simulink model "Ford_T3T6_ArchCnctnDigrm"  (R2016b)
settings: Solver=FixedStepDiscrete  StartTime=0.0  StopTime=10.0  RelTol=1e-3  EnableMultiTasking=on
libraries: canmsglib x15
(part 10 of 15)

== system Ford_T3T6_ArchCnctnDigrm/Monitor System/Measured Signals/ADC ==
  note: ASIL D
  CM012A_FordT3McuCfg : Subsystem  Tag=2.1.0  Description=Program specific I/O and Constant settings for the Ford T3 Program
      settings: AttributesFormatString=Version: %<Tag>
  ES251A_BattRtnCurr : Subsystem  Tag=1.1.0  Description=Receives ADC samples and converts them to battery return current levelexpressed in amperes. Current is saturated before outputed.
      settings: AttributesFormatString=Version: %<Tag>
  EcuT : Outport
  BattVltg : Outport  Port=2
  BattVltgSwd1 : Outport  Port=3
  tag scope: Adc1ScanGroup2Ref0=global, Adc1ScanGroup2Ref1=global, Adc1ScanGroup3Ref0=global, Adc1ScanGroup3Ref1=global, Adc1SelfDiag0=global, Adc1SelfDiag2=global, Adc1SelfDiag4=global, BattRtnCurrAdc=global, BattRtnCurrAdcFaild=global, BattRtnCurrAmpr=global, BattRtnCurrStsQlfr=global, BattVltg=global, BattVltgAdcFaild=global, BattVltgSwd1=global, BattVltgSwd1AdcFaild=global, ChrgPmpDiag=global, ChrgPmpDiagAdcFaild=global, EcuT=global, EcuTAdcFaild=global, HwAg1SnsrNr=global, HwAg1SnsrTyp=global, MotAg2Cos=global, MotAg2CosAdcFaild=global, MotAg2Sin=global, MotAg2SinAdcFaild=global, MotAg5CosAdcFaild=global, MotAg5SinAdcFaild=global, MotAg6CosAdcFaild=global, MotAg6SinAdcFaild=global, MotCtrlAdc0ScanGroup2Ref0=global, MotCtrlAdc0ScanGroup2Ref1=global, MotCtrlAdc0ScanGroup3Ref0=global, MotCtrlAdc0ScanGroup3Ref1=global, MotCtrlAdc0SelfDiag0=global, MotCtrlAdc0SelfDiag2=global, MotCtrlAdc0SelfDiag4=global, MotCtrlBattRtnCurrAmprFastLoop=global, MotCtrlMotAg5Cos=global, MotCtrlMotAg5Sin=global, MotCtrlMotAg6Cos=global, MotCtrlMotAg6Sin=global, MotCtrlMotCurrAdcPeakA=global, MotCtrlMotCurrAdcPeakB=global, MotCtrlMotCurrAdcPeakC=global, MotCtrlMotCurrAdcVlyA=global, MotCtrlMotCurrAdcVlyB=global, MotCtrlMotCurrAdcVlyC=global, MotCtrlMotCurrSnsrOffs1=global, MotCurrAdcPeakAAdcFaild=global, MotCurrAdcPeakBAdcFaild=global, MotCurrAdcPeakCAdcFaild=global, MotCurrAdcVlyAAdcFaild=global, MotCurrAdcVlyBAdcFaild=global, MotCurrAdcVlyCAdcFaild=global, MotCurrSnsrOffs1AdcFaild=global, MotDrvr1IninTestCmpl=global, PwrDiscnctSwtDiag=global, PwrDiscnctSwtDiagAdcFaild=global
  wires:
  [Adc0Faild] -> CM012A_FordT3McuCfg/1(Adc0Faild)
  [Adc1Faild] -> CM012A_FordT3McuCfg/2(Adc1Faild)
  [Adc1RawRes] -> CM012A_FordT3McuCfg/3(Adc1RawRes)
  [EcuId] -> CM012A_FordT3McuCfg/4(EcuId)
  [MotCtrlAdc0RawRes] -> CM012A_FordT3McuCfg/5(MotCtrlAdc0RawRes)
  [GetRefTmr1MicroSec32bit] -> CM012A_FordT3McuCfg/6(GetRefTmr1MicroSec32bit)
  [GetTiSpan1MicroSec32bit] -> CM012A_FordT3McuCfg/7(GetTiSpan1MicroSec32bit)
  CM012A_FordT3McuCfg/1(Adc1ScanGroup2Ref0) -> [Adc1ScanGroup2Ref0]
  CM012A_FordT3McuCfg/2(Adc1ScanGroup2Ref1) -> [Adc1ScanGroup2Ref1]
  CM012A_FordT3McuCfg/3(Adc1ScanGroup3Ref0) -> [Adc1ScanGroup3Ref0]
  CM012A_FordT3McuCfg/4(Adc1ScanGroup3Ref1) -> [Adc1ScanGroup3Ref1]
  CM012A_FordT3McuCfg/5(Adc1SelfDiag0) -> [Adc1SelfDiag0]
  CM012A_FordT3McuCfg/6(Adc1SelfDiag2) -> [Adc1SelfDiag2]
  CM012A_FordT3McuCfg/7(Adc1SelfDiag4) -> [Adc1SelfDiag4]
  CM012A_FordT3McuCfg/8(BattRtnCurrAdc) -> [BattRtnCurrAdc]
  CM012A_FordT3McuCfg/9(BattRtnCurrAdcFaild) -> [BattRtnCurrAdcFaild]
  CM012A_FordT3McuCfg/10(BattVltg) -> BattVltg/1, [BattVltg]
  CM012A_FordT3McuCfg/11(BattVltgAdcFaild) -> [BattVltgAdcFaild]
  CM012A_FordT3McuCfg/12(BattVltgSwd1) -> BattVltgSwd1/1, [BattVltgSwd1]
  CM012A_FordT3McuCfg/13(BattVltgSwd1AdcFaild) -> [BattVltgSwd1AdcFaild]
  CM012A_FordT3McuCfg/14(ChrgPmpDiag) -> [ChrgPmpDiag]
  CM012A_FordT3McuCfg/15(ChrgPmpDiagAdcFaild) -> [ChrgPmpDiagAdcFaild]
  CM012A_FordT3McuCfg/16(EcuT) -> EcuT/1, [EcuT]
  CM012A_FordT3McuCfg/17(EcuTAdcFaild) -> [EcuTAdcFaild]
  CM012A_FordT3McuCfg/18(HwAg1SnsrNr) -> [HwAg1SnsrNr]
  CM012A_FordT3McuCfg/19(HwAg1SnsrTyp) -> [HwAg1SnsrTyp]
  CM012A_FordT3McuCfg/20(MotAg2Cos) -> [MotAg2Cos]
  CM012A_FordT3McuCfg/21(MotAg2CosAdcFaild) -> [MotAg2CosAdcFaild]
  CM012A_FordT3McuCfg/22(MotAg2Sin) -> [MotAg2Sin]
  CM012A_FordT3McuCfg/23(MotAg2SinAdcFaild) -> [MotAg2SinAdcFaild]
  CM012A_FordT3McuCfg/24(MotAg5CosAdcFaild) -> [MotAg5CosAdcFaild]
  CM012A_FordT3McuCfg/25(MotAg5SinAdcFaild) -> [MotAg5SinAdcFaild]
  CM012A_FordT3McuCfg/26(MotAg6CosAdcFaild) -> [MotAg6CosAdcFaild]
  CM012A_FordT3McuCfg/27(MotAg6SinAdcFaild) -> [MotAg6SinAdcFaild]
  CM012A_FordT3McuCfg/28(MotCurrAdcPeakAAdcFaild) -> [MotCurrAdcPeakAAdcFaild]
  CM012A_FordT3McuCfg/29(MotCurrAdcPeakBAdcFaild) -> [MotCurrAdcPeakBAdcFaild]
  CM012A_FordT3McuCfg/30(MotCurrAdcPeakCAdcFaild) -> [MotCurrAdcPeakCAdcFaild]
  CM012A_FordT3McuCfg/31(MotCurrAdcVlyAAdcFaild) -> [MotCurrAdcVlyAAdcFaild]
  CM012A_FordT3McuCfg/32(MotCurrAdcVlyBAdcFaild) -> [MotCurrAdcVlyBAdcFaild]
  CM012A_FordT3McuCfg/33(MotCurrAdcVlyCAdcFaild) -> [MotCurrAdcVlyCAdcFaild]
  CM012A_FordT3McuCfg/34(MotCurrSnsrOffs1AdcFaild) -> [MotCurrSnsrOffs1AdcFaild]
  CM012A_FordT3McuCfg/35(PwrDiscnctSwtDiag) -> [PwrDiscnctSwtDiag]
  CM012A_FordT3McuCfg/36(PwrDiscnctSwtDiagAdcFaild) -> [PwrDiscnctSwtDiagAdcFaild]
  CM012A_FordT3McuCfg/37(MotDrvr1IninTestCmpl) -> [MotDrvr1IninTestCmpl]
  CM012A_FordT3McuCfg/38(MotCtrlAdc0ScanGroup2Ref0) -> [MotCtrlAdc0ScanGroup2Ref0]
  CM012A_FordT3McuCfg/39(MotCtrlAdc0ScanGroup2Ref1) -> [MotCtrlAdc0ScanGroup2Ref1]
  CM012A_FordT3McuCfg/40(MotCtrlAdc0ScanGroup3Ref0) -> [MotCtrlAdc0ScanGroup3Ref0]
  CM012A_FordT3McuCfg/41(MotCtrlAdc0ScanGroup3Ref1) -> [MotCtrlAdc0ScanGroup3Ref1]
  CM012A_FordT3McuCfg/42(MotCtrlAdc0SelfDiag0) -> [MotCtrlAdc0SelfDiag0]
  CM012A_FordT3McuCfg/43(MotCtrlAdc0SelfDiag2) -> [MotCtrlAdc0SelfDiag2]
  CM012A_FordT3McuCfg/44(MotCtrlAdc0SelfDiag4) -> [MotCtrlAdc0SelfDiag4]
  CM012A_FordT3McuCfg/45(MotCtrlMotAg5Cos) -> [MotCtrlMotAg5Cos]
  CM012A_FordT3McuCfg/46(MotCtrlMotAg5Sin) -> [MotCtrlMotAg5Sin]
  CM012A_FordT3McuCfg/47(MotCtrlMotAg6Cos) -> [MotCtrlMotAg6Cos]
  CM012A_FordT3McuCfg/48(MotCtrlMotAg6Sin) -> [MotCtrlMotAg6Sin]
  CM012A_FordT3McuCfg/49(MotCtrlMotCurrAdcPeakA) -> [MotCtrlMotCurrAdcPeakA]
  CM012A_FordT3McuCfg/50(MotCtrlMotCurrAdcPeakB) -> [MotCtrlMotCurrAdcPeakB]
  CM012A_FordT3McuCfg/51(MotCtrlMotCurrAdcPeakC) -> [MotCtrlMotCurrAdcPeakC]
  CM012A_FordT3McuCfg/52(MotCtrlMotCurrAdcVlyA) -> [MotCtrlMotCurrAdcVlyA]
  CM012A_FordT3McuCfg/53(MotCtrlMotCurrAdcVlyB) -> [MotCtrlMotCurrAdcVlyB]
  CM012A_FordT3McuCfg/54(MotCtrlMotCurrAdcVlyC) -> [MotCtrlMotCurrAdcVlyC]
  CM012A_FordT3McuCfg/55(MotCtrlMotCurrSnsrOffs1) -> [MotCtrlMotCurrSnsrOffs1]
  [BattRtnCurrAdc] -> ES251A_BattRtnCurr/1(BattRtnCurrAdc)
  [BattRtnCurrAdcFaild] -> ES251A_BattRtnCurr/2(BattRtnCurrAdcFaild)
  [SplyCurrEstim] -> ES251A_BattRtnCurr/3(SplyCurrEstim)
  [SysSt] -> ES251A_BattRtnCurr/4(SysSt)
  [MotCtrlBattRtnCurrAdc] -> ES251A_BattRtnCurr/5(MotCtrlBattRtnCurrAdc)
  [CnvSnpshtData_f32] -> ES251A_BattRtnCurr/6(CnvSnpshtData_f32)
  [CnvSnpshtData_u08] -> ES251A_BattRtnCurr/7(CnvSnpshtData_u08)
  [GetNtcQlfrSts] -> ES251A_BattRtnCurr/8(GetNtcQlfrSts)
  [SetNtcStsAndSnpshtData] -> ES251A_BattRtnCurr/9(SetNtcStsAndSnpshtData)
  ES251A_BattRtnCurr/1(BattRtnCurrAmpr) -> [BattRtnCurrAmpr]
  ES251A_BattRtnCurr/2(BattRtnCurrStsQlfr) -> [BattRtnCurrStsQlfr]
  ES251A_BattRtnCurr/3(MotCtrlBattRtnCurrAmprFastLoop) -> [MotCtrlBattRtnCurrAmprFastLoop]

== system Ford_T3T6_ArchCnctnDigrm/Monitor System/Measured Signals/BatteryVoltage ==
  note: ASIL B
  note: ASIL B
  BattVltg : Inport
  BattVltgSwd1 : Inport  Port=2
  ES250B_BattVltg : Subsystem  Tag=1.1.0  Description=Function produces an output voltage that is used by the software application
      settings: AttributesFormatString=Version: %<Tag>
  ES259B_BattVltgCorrln : Subsystem  Tag=1.4.0  Description=This function does the correlation between the 2 input sensor signals to determine if they are valid.
      settings: AttributesFormatString=Version: %<Tag>
  Terminator : Terminator
  tag scope: BrdgVltg=global, DftBrdgVltgActv=global, SwdVltgLimd=global
  wires:
  ES259B_BattVltgCorrln/2(BattVltgCorrlnIdptSig) -> Terminator/1
  ES259B_BattVltgCorrln/1(BattSwdVltgCorrlnSts) -> ES250B_BattVltg/1(BattSwdVltgCorrlnSts)
  ES250B_BattVltg/1(BrdgVltg) -> [BrdgVltg]
  BattVltg/1 -> ES259B_BattVltgCorrln/1(BattVltg), ES250B_BattVltg/2(BattVltg)
  BattVltgSwd1/1 -> ES250B_BattVltg/3(BattVltgSwd1), ES259B_BattVltgCorrln/3(BattVltgSwd1)
  [DiagcStsIvtr1Inactv] -> ES259B_BattVltgCorrln/5(DiagcStsIvtr1Inactv)
  [FordInhbBattVltgDiagc] -> ES259B_BattVltgCorrln/6(InhbBattVltgDiagc)
  [StrtUpSt] -> ES259B_BattVltgCorrln/7(StrtUpSt)
  [SysSt] -> ES259B_BattVltgCorrln/8(SysSt)
  [GetNtcQlfrSts8] -> ES259B_BattVltgCorrln/9(GetNtcQlfrSts)
  [SetNtcSts8] -> ES259B_BattVltgCorrln/10(SetNtcSts)
  ES259B_BattVltgCorrln/3(DftBrdgVltgActv) -> [DftBrdgVltgActv]
  ES259B_BattVltgCorrln/4(SwdVltgLimd) -> [SwdVltgLimd]
  [BattVltgSwd1AdcFaild] -> ES259B_BattVltgCorrln/4(BattVltgSwd1AdcFaild)
  [BattVltgAdcFaild] -> ES259B_BattVltgCorrln/2(BattVltgAdcFaild)

== system Ford_T3T6_ArchCnctnDigrm/Monitor System/Measured Signals/EcuTemp ==
  note: ASIL B
  EcuT : Inport
  ES210A_EcuTMeas : Subsystem  Tag=4.2.0  Description="Measures and diagnoses an analog based temperature sensor on ECU.  This particular design can tolerate a transfer function that is not necessarily linear but can be interpolated with 8 different XY pairs."
      settings: AttributesFormatString=Version: %<Tag>
  EcuTFild : Outport
  tag scope: DiagcStsLimdTPrfmnc=global, EcuTFild=global
  wires:
  EcuT/1 -> ES210A_EcuTMeas/1(EcuT)
  [EcuTAdcFaild] -> ES210A_EcuTMeas/2(EcuTAdcFaild)
  [CnvSnpshtData_f32] -> ES210A_EcuTMeas/3(CnvSnpshtData_f32)
  [CnvSnpshtData_logl] -> ES210A_EcuTMeas/4(CnvSnpshtData_logl)
  [GetNtcActv8] -> ES210A_EcuTMeas/5(GetNtcActv)
  [SetNtcStsAndSnpshtData8] -> ES210A_EcuTMeas/6(SetNtcStsAndSnpshtData)
  ES210A_EcuTMeas/1(DiagcStsLimdTPrfmnc) -> [DiagcStsLimdTPrfmnc]
  ES210A_EcuTMeas/2(EcuTFild) -> EcuTFild/1, [EcuTFild]

== system Ford_T3T6_ArchCnctnDigrm/Monitor System/Measured Signals/HwAg Signal Measurement and  Arbitration ==
  note: ASIL D
  note: ASIL D
  note: ASIL D
  CM670A_HwAg1Meas : Subsystem  Tag=3.2.1  Description=HandWheel Angle Sensor 1 Measurement Function reads 10th Tooth and 11th Tooth Spur Handwheel angles over SENT and compute absolute Handwheel Angle 1. Function also provides Fault Injection and Trim Manufacturing services
      settings: AttributesFormatString=Version: %<Tag>
  ES238A_HwAgArbn : Subsystem  Tag=2.2.0  Description=Arbitrates handwheel angle channels and provides handwheel angle to the application
      settings: AttributesFormatString=Version: %<Tag>
  ES239A_HwAgCorrln : Subsystem  Tag=2.2.0  Description=Provides signal correlation for handwheel angle per the SSI design.
      settings: AttributesFormatString=Version: %<Tag>
  HwAgMeas : Outport
  HwAgIdptSig : Outport  Port=2
  tag scope: HwAg1AutTrim=global, HwAg1ClrLtch=global, HwAg1ClrTrim=global, HwAg1ReadTrim=global, HwAg1TrimPrfmdSts=global, HwAg1WrTrim=global, HwAgMeas=global
  wires:
  [HwAgAPolarity] -> CM670A_HwAg1Meas/1(HwAg1Polarity)
  [HwAg1SnsrTyp] -> CM670A_HwAg1Meas/2(HwAg1SnsrTyp)
  [CnvSnpshtData_f32] -> CM670A_HwAg1Meas/3(CnvSnpshtData_f32)
  [CnvSnpshtData_u08] -> CM670A_HwAg1Meas/4(CnvSnpshtData_u08)
  [FltInj_u08] -> CM670A_HwAg1Meas/5(FltInj_u08)
  [GetNtcQlfrSts] -> CM670A_HwAg1Meas/6(GetNtcQlfrSts)
  [GetRefTmr1MicroSec32bit] -> CM670A_HwAg1Meas/7(GetRefTmr1MicroSec32bit)
  [GetTiSpan1MicroSec32bit] -> CM670A_HwAg1Meas/8(GetTiSpan1MicroSec32bit)
  [NvMProxy_GetErrorStatus] -> CM670A_HwAg1Meas/9(HwAg1IfFltLtch_GetErrorStatus)
  [NvMProxy_SetRamBlockStatus] -> CM670A_HwAg1Meas/10(HwAg1IfFltLtch_SetRamBlockStatus)
  [NvMProxy_GetErrorStatus] -> CM670A_HwAg1Meas/11(HwAg1Offs_GetErrorStatus)
  [NvMProxy_SetRamBlockStatus] -> CM670A_HwAg1Meas/12(HwAg1Offs_SetRamBlockStatus)
  [IoHwAb_SetFctPrphlHwAg1] -> CM670A_HwAg1Meas/13(IoHwAb_SetFctPrphlHwAg1)
  [SetNtcStsAndSnpshtData10] -> CM670A_HwAg1Meas/14(SetNtcStsAndSnpshtData)
  CM670A_HwAg1Meas/4(HwAg1AutTrim) -> [HwAg1AutTrim]
  CM670A_HwAg1Meas/5(HwAg1ClrLtch) -> [HwAg1ClrLtch]
  CM670A_HwAg1Meas/6(HwAg1ClrTrim) -> [HwAg1ClrTrim]
  CM670A_HwAg1Meas/7(HwAg1ReadTrim) -> [HwAg1ReadTrim]
  CM670A_HwAg1Meas/8(HwAg1TrimPrfmdSts) -> [HwAg1TrimPrfmdSts]
  CM670A_HwAg1Meas/9(HwAg1WrTrim) -> [HwAg1WrTrim]
  CM670A_HwAg1Meas/3(HwAg1RollgCntr) -> ES238A_HwAgArbn/3(HwAgAQlfr), ES239A_HwAgCorrln/4(HwAgARollgCntr)
  [HwAgARollgCntr] -> ES238A_HwAgArbn/4(HwAgARollgCntr)
  [HwAgB] -> ES238A_HwAgArbn/5(HwAgB)
  [HwAgBQlfr] -> ES238A_HwAgArbn/6(HwAgBQlfr)
  [HwAgBRollgCntr] -> ES238A_HwAgArbn/7(HwAgBRollgCntr)
  [FltInj_f32] -> ES238A_HwAgArbn/9(FltInj_f32)
  ES238A_HwAgArbn/1(HwAg) -> HwAgMeas/1, [HwAgMeas]
  [HwAg1SnsrNr] -> ES239A_HwAgCorrln/1(HwAg1SnsrNr)
  CM670A_HwAg1Meas/1(HwAg1) -> ES238A_HwAgArbn/1(HwAg1SnsrNr), ES239A_HwAgCorrln/2(HwAgA)
  CM670A_HwAg1Meas/2(HwAg1Qlfr) -> ES238A_HwAgArbn/2(HwAgA), ES239A_HwAgCorrln/3(HwAgAQlfr)
  [HwAgB] -> ES239A_HwAgCorrln/5(HwAgB)
  [HwAgBQlfr] -> ES239A_HwAgCorrln/6(HwAgBQlfr)
  [HwAgBRollgCntr] -> ES239A_HwAgCorrln/7(HwAgBRollgCntr)
  [FltInj_u08] -> ES239A_HwAgCorrln/8(FltInj_u08)
  [GetNtcQlfrSts] -> ES239A_HwAgCorrln/9(GetNtcQlfrSts)
  [SetNtcSts] -> ES239A_HwAgCorrln/10(SetNtcSts)
  ES239A_HwAgCorrln/1(HwAgCorrlnSt) -> ES238A_HwAgArbn/8(HwAgCorrlnSt)
  ES239A_HwAgCorrln/2(HwAgIdptSig) -> HwAgIdptSig/1

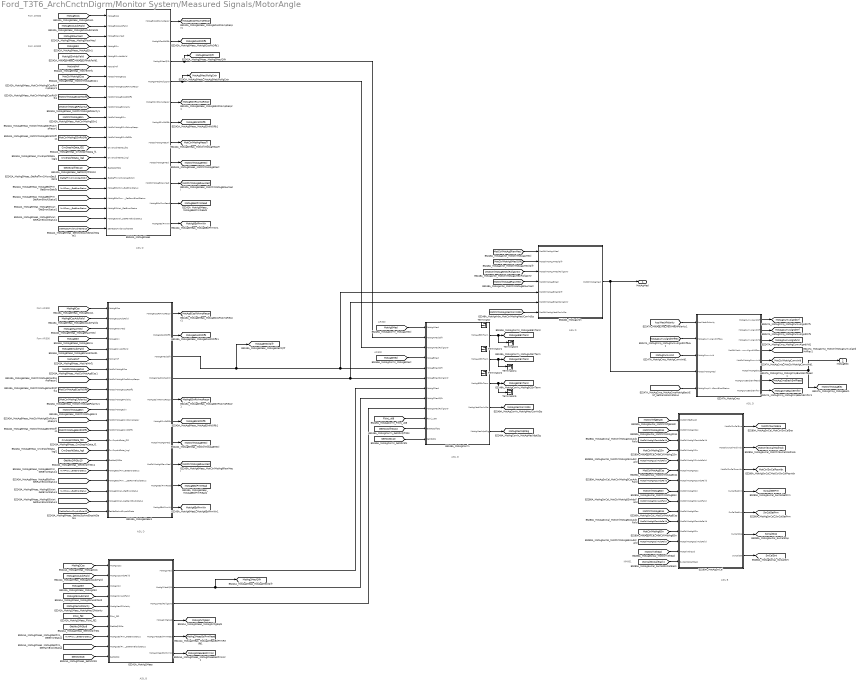
== system Ford_T3T6_ArchCnctnDigrm/Monitor System/Measured Signals/MotorAngle ==
  note: AR300
  note: Fom AR300
  note: ASIL D
  note: ASIL D
  note: ASIL B
  note: ASIL D
  note: ASIL D
  note: ASIL D
  note: ASIL B
  note: Fom AR300
  note: Fom AR300
  note: Fom AR300
  note: AR300
  note: NM001
  ES241A_MotAg2Meas : Subsystem  Tag=1.10.0  Description=This function is responsible for providing a qualified, tertiary motor angle measurement using a sine / cosine based analog sensor
      settings: AttributesFormatString=Version: %<Tag>
  ES242A_MotAg5Meas : Subsystem  Tag=1.3.0  Description=MotAg5Meas funtion shall compute motor angle from Sine and Cosine ADC signals
      settings: AttributesFormatString=Version: %<Tag>
  ES243A_MotAg6Meas1 : Subsystem  Tag=1.4.0  Description=MotAg6Meas funtion shall compute motor angle from Sine and Cosine ADC signals
      settings: AttributesFormatString=Version: %<Tag>
  ES247A_MotAgCmp : Subsystem  Tag=1.8.0  Description=Compensates motor angle for Back EMF and computes cumulative position
      settings: AttributesFormatString=Version: %<Tag>
  ES248A_MotAgArbn : Subsystem  Tag=1.3.0  Description="This function will arbitrate between to motor angle measurements in the motor control loop.  This design assumes that motor angle A is the primary sensor and will use it when possible."
      settings: AttributesFormatString=Version: %<Tag>
  ES249A_MotAgCorrln : Subsystem  Tag=5.0.0  Description=Performs cross check of available motor angle signals. This is necessary for the loss of assist mitigation strategies
      settings: AttributesFormatString=Version: %<Tag>
  ES280A_MotAgSwCal : Subsystem  Tag=2.1.0  Description=Motor Angle Software Calibration
      settings: AttributesFormatString=Version: %<Tag>
  Terminator{,1..5} (6 alike) : Terminator
  MotAgMecl : Outport
  MotAgElec : Outport  Port=2
  tag scope: MotAg2MeasEolPrmRead=global, MotAg2MeasEolPrmWr=global, MotAg2MeclQlfr=global, MotAg2VltgSqd=global, MotAg5CosRtAmpRecpr=global, MotAg5CosRtOffs=global, MotAg5EolPrmRead=global, MotAg5EolPrmWr=global, MotAg5MeclQlfr=global, MotAg5MeclRollgCntr=global, MotAg5SinRtAmpRecpr=global, MotAg5SinRtOffs=global, MotAg6CosRtAmpRecpr=global, MotAg6CosRtOffs=global, MotAg6EolPrmRead=global, MotAg6EolPrmWr=global, MotAg6MeclQlfr=global, MotAg6SinRtAmpRecpr=global, MotAg6SinRtOffs=global, MotAgABErrTerm=global, MotAgACErrTerm=global, MotAgBCErrTerm=global, MotAgCmpBackEmfRead=global, MotAgCmpBackEmfWr=global, MotAgCumvAlgndCrf=global, MotAgCumvAlgndMrf=global, MotAgCumvAlgndVld=global, MotAgMeclCorrlnSts=global, MotAgMeclIdptSig=global, MotCtrlMotAg5Mecl=global, MotCtrlMotAg5RawMecl=global, MotCtrlMotAg6Mecl=global, MotCtrlMotAg6RawMecl=global, MotCtrlMotAgCumvAlgndMrfRev=global, MotCtrlMotAgCumvInid=global, MotCtrlMotAgElec=global, MotCtrlMotAgMeasTi=global, MotCtrlSwCalEna=global, MotCtrlSwCalModlnIdx=global, MotCtrlSwCalPosnIdx=global, SwCalGetPrm=global, SwCalSetPrm=global, SwCalStop=global, SwCalStrt=global
  wires:
  ES247A_MotAgCmp/6(MotCtrlMotAgElec) -> MotAgElec/1, [MotCtrlMotAgElec]
  ES243A_MotAg6Meas1/3(MotAg6MeclQlfr) -> [MotAg6MeclQlfr], ES249A_MotAgCorrln/5(MotAgBMeclQlfr), ES248A_MotAgArbn/5(MotCtrlMotAgBMeclQlfr)
  ES243A_MotAg6Meas1/4(MotAg6MeclRollgCntr) -> ES249A_MotAgCorrln/6(MotAgBMeclRollgCntr), ES248A_MotAgArbn/6(MotCtrlMotAgBMeclRollgCntr)
  ES242A_MotAg5Meas/4(MotAg5MeclRollgCntr) -> [MotAg5MeclRollgCntr], ES249A_MotAgCorrln/3(MotAgAMeclRollgCntr)
  ES242A_MotAg5Meas/3(MotAg5MeclQlfr) -> [MotAg5MeclQlfr], ES249A_MotAgCorrln/2(MotAgAMeclQlfr)
  ES241A_MotAg2Meas/1(MotAg2Mecl) -> ES249A_MotAgCorrln/7(MotAgCMecl)
  ES241A_MotAg2Meas/2(MotAg2MeclQlfr) -> [MotAg2MeclQlfr], ES249A_MotAgCorrln/8(MotAgCMeclQlfr)
  ES241A_MotAg2Meas/3(MotAg2MeclRollgCntr) -> ES249A_MotAgCorrln/9(MotAgCMeclRollgCntr)
  [MotCtrlMfgEnaSt] -> ES280A_MotAgSwCal/1(MotCtrlMfgEnaSt)
  [MotCtrlMotAg2Cos] -> ES280A_MotAgSwCal/2(MotCtrlMotAg2Cos)
  [MotCtrlMotAg2CosAdcFaild] -> ES280A_MotAgSwCal/3(MotCtrlMotAg2CosAdcFaild)
  [MotCtrlMotAg2Sin] -> ES280A_MotAgSwCal/4(MotCtrlMotAg2Sin)
  [MotCtrlMotAg2SinAdcFaild] -> ES280A_MotAgSwCal/5(MotCtrlMotAg2SinAdcFaild)
  [MotCtrlMotAg5Cos] -> ES280A_MotAgSwCal/6(MotCtrlMotAg5Cos)
  [MotCtrlMotAg5CosAdcFaild] -> ES280A_MotAgSwCal/7(MotCtrlMotAg5CosAdcFaild)
  [MotCtrlMotAg5Sin] -> ES280A_MotAgSwCal/8(MotCtrlMotAg5Sin)
  [MotCtrlMotAg5SinAdcFaild] -> ES280A_MotAgSwCal/9(MotCtrlMotAg5SinAdcFaild)
  [MotCtrlMotAg6Cos] -> ES280A_MotAgSwCal/10(MotCtrlMotAg6Cos)
  [MotCtrlMotAg6CosAdcFaild] -> ES280A_MotAgSwCal/11(MotCtrlMotAg6CosAdcFaild)
  [MotCtrlMotAg6Sin] -> ES280A_MotAgSwCal/12(MotCtrlMotAg6Sin)
  [MotCtrlMotAg6SinAdcFaild] -> ES280A_MotAgSwCal/13(MotCtrlMotAg6SinAdcFaild)
  [MotCtrlVehSpd] -> ES280A_MotAgSwCal/14(MotCtrlVehSpd)
  [SwCalStsCallBack] -> ES280A_MotAgSwCal/15(SwCalStsCallBack)
  ES280A_MotAgSwCal/1(MotCtrlSwCalEna) -> [MotCtrlSwCalEna]
  ES280A_MotAgSwCal/2(MotCtrlSwCalModlnIdx) -> [MotCtrlSwCalModlnIdx]
  ES280A_MotAgSwCal/3(MotCtrlSwCalPosnIdx) -> [MotCtrlSwCalPosnIdx]
  ES280A_MotAgSwCal/4(SwCalGetPrm) -> [SwCalGetPrm]
  ES280A_MotAgSwCal/5(SwCalSetPrm) -> [SwCalSetPrm]
  ES280A_MotAgSwCal/6(SwCalStop) -> [SwCalStop]
  ES280A_MotAgSwCal/7(SwCalStrt) -> [SwCalStrt]
  [FltInj_u08] -> ES249A_MotAgCorrln/10(FltInj_u08)
  [GetNtcQlfrSts10] -> ES249A_MotAgCorrln/11(GetNtcQlfrSts)
  [SetNtcSts10] -> ES249A_MotAgCorrln/12(SetNtcSts)
  ES249A_MotAgCorrln/1(MotAgABErrTerm) -> Terminator3/1, [MotAgABErrTerm]
  ES249A_MotAgCorrln/2(MotAgACErrTerm) -> Terminator4/1, [MotAgACErrTerm]
  ES249A_MotAgCorrln/3(MotAgBCErrTerm) -> Terminator5/1, [MotAgBCErrTerm]
  ES249A_MotAgCorrln/5(MotAgMeclIdptSig) -> [MotAgMeclIdptSig]
  [MotAg2Cos] -> ES241A_MotAg2Meas/1(MotAg2Cos)
  [MotAg2CosAdcFaild] -> ES241A_MotAg2Meas/2(MotAg2CosAdcFaild)
  [MotAg2Sin] -> ES241A_MotAg2Meas/3(MotAg2Sin)
  [MotAg2SinAdcFaild] -> ES241A_MotAg2Meas/4(MotAg2SinAdcFaild)
  [MotAgMeclAPolarity] -> ES241A_MotAg2Meas/5(MotAgMecl2Polarity)
  [FltInj_f32] -> ES241A_MotAg2Meas/6(FltInj_f32)
  [GetNtcQlfrSts8] -> ES241A_MotAg2Meas/7(GetNtcQlfrSts)
  [NvMProxy_GetErrorStatus] -> ES241A_MotAg2Meas/8(MotAg2EolPrm_GetErrorStatus)
  [NvMProxy_SetRamBlockStatus] -> ES241A_MotAg2Meas/9(MotAg2EolPrm_SetRamBlockStatus)
  [SetNtcSts8] -> ES241A_MotAg2Meas/10(SetNtcSts)
  ES241A_MotAg2Meas/4(MotAg2VltgSqd) -> [MotAg2VltgSqd]
  ES241A_MotAg2Meas/5(MotAg2MeasEolPrmRead) -> [MotAg2MeasEolPrmRead]
  ES241A_MotAg2Meas/6(MotAg2MeasEolPrmWr) -> [MotAg2MeasEolPrmWr]
  [MotAg5Cos] -> ES242A_MotAg5Meas/1(MotAg5Cos)
  [MotAg5CosAdcFaild] -> ES242A_MotAg5Meas/2(MotAg5CosAdcFaild)
  [MotAg0RawMecl] -> ES242A_MotAg5Meas/3(MotAg5RawMecl)
  [MotAg5Sin] -> ES242A_MotAg5Meas/4(MotAg5Sin)
  [MotAg5SinAdcFaild] -> ES242A_MotAg5Meas/5(MotAg5SinAdcFaild)
  [MotVelMrf] -> ES242A_MotAg5Meas/6(MotVelMrf)
  [MotCtrlMotAg5Cos] -> ES242A_MotAg5Meas/7(MotCtrlMotAg5Cos)
  [MotCtrlMotAg5CosRtAmpRecpr] -> ES242A_MotAg5Meas/8(MotCtrlMotAg5CosRtAmpRecpr)
  [MotCtrlMotAg5CosRtOffs] -> ES242A_MotAg5Meas/9(MotCtrlMotAg5CosRtOffs)
  [MotCtrlMotAgBPolarity] -> ES242A_MotAg5Meas/10(MotCtrlMotAg5Polarity)
  [MotCtrlMotAg5Sin] -> ES242A_MotAg5Meas/11(MotCtrlMotAg5Sin)
  [MotCtrlMotAg5SinRtAmpRecpr] -> ES242A_MotAg5Meas/12(MotCtrlMotAg5SinRtAmpRecpr)
  [MotCtrlMotAg5SinRtOffs] -> ES242A_MotAg5Meas/13(MotCtrlMotAg5SinRtOffs)
  [CnvSnpshtData_f32] -> ES242A_MotAg5Meas/14(CnvSnpshtData_f32)
  [CnvSnpshtData_logl] -> ES242A_MotAg5Meas/15(CnvSnpshtData_logl)
  [GetNtcQlfrSts10] -> ES242A_MotAg5Meas/16(GetNtcQlfrSts)
  [GetRefTmr1MicroSec32bit] -> ES242A_MotAg5Meas/17(GetRefTmr1MicroSec32bit)
  [NvMProxy_GetErrorStatus] -> ES242A_MotAg5Meas/18(MotAg5EolPrm_GetErrorStatus)
  [NvMProxy_SetRamBlockStatus] -> ES242A_MotAg5Meas/19(MotAg5EolPrm_SetRamBlockStatus)
  [NvMProxy_GetErrorStatus] -> ES242A_MotAg5Meas/20(MotAg5StVari_GetErrorStatus)
  [NvMProxy_SetRamBlockStatus] -> ES242A_MotAg5Meas/21(MotAg5StVari_SetRamBlockStatus)
  [SetNtcStsAndSnpshtData10] -> ES242A_MotAg5Meas/22(SetNtcStsAndSnpshtData)
  ES242A_MotAg5Meas/1(MotAg5CosRtAmpRecpr) -> [MotAg5CosRtAmpRecpr]
  ES242A_MotAg5Meas/2(MotAg5CosRtOffs) -> [MotAg5CosRtOffs]
  ES242A_MotAg5Meas/5(MotAg5SinRtAmpRecpr) -> [MotAg5SinRtAmpRecpr]
  ES242A_MotAg5Meas/6(MotAg5SinRtOffs) -> [MotAg5SinRtOffs]
  ES242A_MotAg5Meas/7(MotCtrlMotAgMeasTi) -> [MotCtrlMotAgMeasTi]
  ES242A_MotAg5Meas/8(MotCtrlMotAg5Mecl) -> [MotCtrlMotAg5Mecl]
  ES242A_MotAg5Meas/10(MotAg5EolPrmRead) -> [MotAg5EolPrmRead]
  ES242A_MotAg5Meas/11(MotAg5EolPrmWr) -> [MotAg5EolPrmWr]
  [MotAg6Cos] -> ES243A_MotAg6Meas1/1(MotAg6Cos)
  [MotAg6CosAdcFaild] -> ES243A_MotAg6Meas1/2(MotAg6CosAdcFaild)
  [MotAg1RawMecl] -> ES243A_MotAg6Meas1/3(MotAg6RawMecl)
  [MotAg6Sin] -> ES243A_MotAg6Meas1/4(MotAg6Sin)
  [MotAg6SinAdcFaild] -> ES243A_MotAg6Meas1/5(MotAg6SinAdcFaild)
  [MotVelMrf] -> ES243A_MotAg6Meas1/6(MotVelMrf)
  [MotCtrlMotAg6Cos] -> ES243A_MotAg6Meas1/7(MotCtrlMotAg6Cos)
  [MotCtrlMotAg6CosRtAmpRecpr] -> ES243A_MotAg6Meas1/8(MotCtrlMotAg6CosRtAmpRecpr)
  [MotCtrlMotAg6CosRtOffs] -> ES243A_MotAg6Meas1/9(MotCtrlMotAg6CosRtOffs)
  [MotCtrlMotAgCPolarity] -> ES243A_MotAg6Meas1/10(MotCtrlMotAg6Polarity)
  [MotCtrlMotAg6Sin] -> ES243A_MotAg6Meas1/11(MotCtrlMotAg6Sin)
  [MotCtrlMotAg6SinRtAmpRecpr] -> ES243A_MotAg6Meas1/12(MotCtrlMotAg6SinRtAmpRecpr)
  [MotCtrlMotAg6SinRtOffs] -> ES243A_MotAg6Meas1/13(MotCtrlMotAg6SinRtOffs)
  [CnvSnpshtData_f32] -> ES243A_MotAg6Meas1/14(CnvSnpshtData_f32)
  [CnvSnpshtData_logl] -> ES243A_MotAg6Meas1/15(CnvSnpshtData_logl)
  [GetNtcQlfrSts10] -> ES243A_MotAg6Meas1/16(GetNtcQlfrSts)
  [NvMProxy_GetErrorStatus] -> ES243A_MotAg6Meas1/17(MotAg6EolPrm_GetErrorStatus)
  [NvMProxy_SetRamBlockStatus] -> ES243A_MotAg6Meas1/18(MotAg6EolPrm_SetRamBlockStatus)
  [NvMProxy_GetErrorStatus] -> ES243A_MotAg6Meas1/19(MotAg6StVari_GetErrorStatus)
  [NvMProxy_SetRamBlockStatus] -> ES243A_MotAg6Meas1/20(MotAg6StVari_SetRamBlockStatus)
  [SetNtcStsAndSnpshtData10] -> ES243A_MotAg6Meas1/21(SetNtcStsAndSnpshtData)
  ES243A_MotAg6Meas1/1(MotAg6CosRtAmpRecpr) -> [MotAg6CosRtAmpRecpr]
  ES243A_MotAg6Meas1/2(MotAg6CosRtOffs) -> [MotAg6CosRtOffs]
  ES243A_MotAg6Meas1/5(MotAg6SinRtAmpRecpr) -> [MotAg6SinRtAmpRecpr]
  ES243A_MotAg6Meas1/6(MotAg6SinRtOffs) -> [MotAg6SinRtOffs]
  ES243A_MotAg6Meas1/7(MotCtrlMotAg6Mecl) -> [MotCtrlMotAg6Mecl]
  ES243A_MotAg6Meas1/9(MotAg6EolPrmRead) -> [MotAg6EolPrmRead]
  ES243A_MotAg6Meas1/10(MotAg6EolPrmWr) -> [MotAg6EolPrmWr]
  [AssiMechPolarity] -> ES247A_MotAgCmp/1(AssiMechPolarity)
  [MotAgCumvAlgndMrfRev] -> ES247A_MotAgCmp/2(MotAgCumvAlgndMrfRev)
  [MotAgCumvInid] -> ES247A_MotAgCmp/3(MotAgCumvInid)
  ES248A_MotAgArbn/1(MotCtrlMotAgMecl) -> ES247A_MotAgCmp/4(MotCtrlMotAgMecl), MotAgMecl/1
  [NvMProxy_SetRamBlockStatus] -> ES247A_MotAgCmp/5(MotAgCmpMotAgBackEmf_SetRamBlockStatus)
  ES247A_MotAgCmp/1(MotAgCumvAlgndCrf) -> [MotAgCumvAlgndCrf]
  ES247A_MotAgCmp/2(MotAgCumvAlgndMrf) -> [MotAgCumvAlgndMrf]
  ES247A_MotAgCmp/3(MotAgCumvAlgndVld) -> [MotAgCumvAlgndVld]
  ES247A_MotAgCmp/4(MotCtrlMotAgCumvAlgndMrfRev) -> [MotCtrlMotAgCumvAlgndMrfRev]
  ES247A_MotAgCmp/5(MotCtrlMotAgCumvInid) -> [MotCtrlMotAgCumvInid]
  ES247A_MotAgCmp/7(MotAgCmpBackEmfRead) -> [MotAgCmpBackEmfRead]
  ES247A_MotAgCmp/8(MotAgCmpBackEmfWr) -> [MotAgCmpBackEmfWr]
  ES249A_MotAgCorrln/4(MotAgMeclCorrlnSts) -> [MotAgMeclCorrlnSts]
  [MotCtrlMotAgMeclCorrlnSts] -> ES248A_MotAgArbn/7(MotCtrlMotAgMeclCorrlnSts)
  ES243A_MotAg6Meas1/8(MotCtrlMotAg6RawMecl) -> [MotCtrlMotAg6RawMecl]
  [MotCtrlMotAg6RawMecl] -> ES248A_MotAgArbn/4(MotCtrlMotAgBMecl)
  [MotAg6Mecl] -> ES249A_MotAgCorrln/4(MotAgBMecl)
  [MotAg5Mecl] -> ES249A_MotAgCorrln/1(MotAgAMecl)
  [MotCtrlMotAg5RawMecl] -> ES248A_MotAgArbn/1(MotCtrlMotAgAMecl)
  [MotCtrlMotAg5MeclQlfr] -> ES248A_MotAgArbn/2(MotCtrlMotAgAMeclQlfr)
  [MotCtrlMotAg5MeclRollgCntr] -> ES248A_MotAgArbn/3(MotCtrlMotAgAMeclRollgCntr)
  ES242A_MotAg5Meas/9(MotCtrlMotAg5RawMecl) -> [MotCtrlMotAg5RawMecl]

== system Ford_T3T6_ArchCnctnDigrm/Monitor System/Measured Signals/MotorCurrent ==
  note: ASIL D
  note: ASIL D
  note: ASIL D
  MotVelMrf : Inport
  MotAgElec : Inport  Port=2
  ES200B_CurrMeas : Subsystem  Tag=2.2.0  Description=The Current Measurement function is responsible for measuring the motor phase currents used as feedback by the Motor Control FDD. Three motor phase currents are measured using three low-side shunt resistors and three integrated differential amplifier circuitry for each motor. Then measured currents are transformed into direct (D) and quadrature (Q) axes currents using the combined Clarke/Park transform.
      settings: AttributesFormatString=Version: %<Tag>
  ES208A_CurrMeasArbn : Subsystem  Tag=1.3.0  Description=The Current Measurement Arbitration function is responsible to selecta sensor value and determine the quality of that sensor value
      settings: AttributesFormatString=Version: %<Tag>
  ES209B_CurrMeasCorrln : Subsystem  Tag=1.7.0  Description=The Current Measurement Correlation function is responsible to determine any correlation fault between signals or channels and to determine the number of independent signals available to use
      settings: AttributesFormatString=Version: %<Tag>
  Ground{,1..4} (5 alike) : Ground
  tag scope: CurrMeasCorrlnSts=global, CurrMeasEolGainReq=global, CurrMeasEolGainStsReq=global, CurrMeasEolOffsReq=global, CurrMeasEolOffsStsReq=global, CurrMeasGainReadReqSngIvtr=global, CurrMeasGainWrReqSngIvtr=global, CurrMeasIdptSig=global, CurrMeasOffsReadReqSngIvtr=global, CurrMeasOffsWrReqSngIvtr=global, CurrMeasWrmIninTestCmpl=global, CurrMotSumABC=global, MotCtrlCurrMeasMotAgCorrd=global, MotCtrlMotCurrDax=global, MotCtrlMotCurrQax=global, MotCtrlNtc5DErrCnt=global, MotCurrEolCalSt=global, MotCurrQlfr1=global
  wires:
  [MotCtrlCurrMeasMotAgCorrd] -> ES208A_CurrMeasArbn/2(MotCtrlCurrMeasMotAgCorrd)
  [MotCurrQlfr1] -> ES208A_CurrMeasArbn/9(MotCtrlMotCurrQlfr1)
  [MotElecMeclPolarity] -> ES208A_CurrMeasArbn/13(MotCtrlMotElecMeclPolarity)
  ES209B_CurrMeasCorrln/1(CurrMeasCorrlnSts) -> [CurrMeasCorrlnSts], ES208A_CurrMeasArbn/1(MotCtrlCurrMeasCorrlnSts)
  ES208A_CurrMeasArbn/2(MotCtrlMotCurrQax) -> [MotCtrlMotCurrQax]
  ES208A_CurrMeasArbn/1(MotCtrlMotCurrDax) -> [MotCtrlMotCurrDax]
  Ground/1 -> ES208A_CurrMeasArbn/6(MotCtrlMotCurrCorrdD)
  Ground1/1 -> ES208A_CurrMeasArbn/7(MotCtrlMotCurrCorrdE)
  Ground2/1 -> ES208A_CurrMeasArbn/8(MotCtrlMotCurrCorrdF)
  Ground3/1 -> ES208A_CurrMeasArbn/10(MotCtrlMotCurrQlfr2)
  Ground4/1 -> ES208A_CurrMeasArbn/12(MotCtrlMotCurrRollgCntr2)
  [BrdgVltg] -> ES200B_CurrMeas/1(BrdgVltg)
  [DiagcStsIvtr1Inactv] -> ES200B_CurrMeas/2(DiagcStsIvtr1Inactv)
  [MotCurrAdcVlyA] -> ES200B_CurrMeas/3(MotCurrAdcVlyA)
  [MotCurrAdcVlyB] -> ES200B_CurrMeas/4(MotCurrAdcVlyB)
  [MotCurrAdcVlyC] -> ES200B_CurrMeas/5(MotCurrAdcVlyC)
  MotVelMrf/1 -> ES200B_CurrMeas/6(MotVelMrf)
  [Ntc5DErrCnt] -> ES200B_CurrMeas/7(Ntc5DErrCnt)
  [StrtUpSt] -> ES200B_CurrMeas/8(StrtUpSt)
  [SysSt] -> ES200B_CurrMeas/9(SysSt)
  [VehSpd] -> ES200B_CurrMeas/10(VehSpd)
  [VehSpdVld] -> ES200B_CurrMeas/11(VehSpdVld)
  [MotCtrlBrdgVltg] -> ES200B_CurrMeas/12(MotCtrlBrdgVltg)
  [MotCtrlCurrMeasWrmIninTestCmpl] -> ES200B_CurrMeas/13(MotCtrlCurrMeasWrmIninTestCmpl)
  [MotCtrlDiagcStsIvtr1Inactv] -> ES200B_CurrMeas/14(MotCtrlDiagcStsIvtr1Inactv)
  [MotCtrlEcuTFild] -> ES200B_CurrMeas/15(MotCtrlEcuTFild)
  MotAgElec/1 -> ES200B_CurrMeas/16(MotCtrlMotAgElec)
  [MotCtrlMotCurrAdcVlyA] -> ES200B_CurrMeas/17(MotCtrlMotCurrAdcVlyA)
  [MotCtrlMotCurrAdcVlyAAdcFaild] -> ES200B_CurrMeas/18(MotCtrlMotCurrAdcVlyAAdcFaild)
  [MotCtrlMotCurrAdcVlyB] -> ES200B_CurrMeas/19(MotCtrlMotCurrAdcVlyB)
  [MotCtrlMotCurrAdcVlyBAdcFaild] -> ES200B_CurrMeas/20(MotCtrlMotCurrAdcVlyBAdcFaild)
  [MotCtrlMotCurrAdcVlyC] -> ES200B_CurrMeas/21(MotCtrlMotCurrAdcVlyC)
  [MotCtrlMotCurrAdcVlyCAdcFaild] -> ES200B_CurrMeas/22(MotCtrlMotCurrAdcVlyCAdcFaild)
  [MotCtrlMotElecMeclPolarity] -> ES200B_CurrMeas/23(MotCtrlMotElecMeclPolarity)
  [MotCtrlMotVelMrf] -> ES200B_CurrMeas/24(MotCtrlMotVelMrf)
  [MotCtrlPhaOnTiA] -> ES200B_CurrMeas/25(MotCtrlPhaOnTiA)
  [MotCtrlPhaOnTiB] -> ES200B_CurrMeas/26(MotCtrlPhaOnTiB)
  [MotCtrlPhaOnTiC] -> ES200B_CurrMeas/27(MotCtrlPhaOnTiC)
  [MotCtrlPwmPerd] -> ES200B_CurrMeas/28(MotCtrlPwmPerd)
  [MotCtrlSysSt] -> ES200B_CurrMeas/29(MotCtrlSysSt)
  [NvMProxy_GetErrorStatus] -> ES200B_CurrMeas/30(CurrMeasEolGainCalSetABC_GetErrorStatus)
  [NvMProxy_SetRamBlockStatus] -> ES200B_CurrMeas/31(CurrMeasEolGainCalSetABC_SetRamBlockStatus)
  [NvMProxy_GetErrorStatus] -> ES200B_CurrMeas/32(CurrMeasEolOffsCalSetABC_GetErrorStatus)
  [NvMProxy_SetRamBlockStatus] -> ES200B_CurrMeas/33(CurrMeasEolOffsCalSetABC_SetRamBlockStatus)
  [FltInj_f32] -> ES200B_CurrMeas/34(FltInj_f32)
  [FltInj_u08] -> ES200B_CurrMeas/35(FltInj_u08)
  [GetNtcQlfrSts10] -> ES200B_CurrMeas/36(GetNtcQlfrSts)
  [SetNtcSts10] -> ES200B_CurrMeas/37(SetNtcSts)
  ES200B_CurrMeas/1(CurrMeasWrmIninTestCmpl) -> [CurrMeasWrmIninTestCmpl]
  ES200B_CurrMeas/2(MotCurrEolCalSt) -> [MotCurrEolCalSt]
  ES200B_CurrMeas/3(MotCurrQlfr1) -> [MotCurrQlfr1]
  ES200B_CurrMeas/4(MotCtrlCurrMeasMotAgCorrd) -> [MotCtrlCurrMeasMotAgCorrd]
  ES200B_CurrMeas/9(MotCtrlNtc5DErrCnt) -> [MotCtrlNtc5DErrCnt]
  ES200B_CurrMeas/10(CurrMeasEolGainReq) -> [CurrMeasEolGainReq]
  ES200B_CurrMeas/11(CurrMeasEolGainStsReq) -> [CurrMeasEolGainStsReq]
  ES200B_CurrMeas/12(CurrMeasEolOffsReq) -> [CurrMeasEolOffsReq]
  ES200B_CurrMeas/13(CurrMeasEolOffsStsReq) -> [CurrMeasEolOffsStsReq]
  ES200B_CurrMeas/14(CurrMeasGainReadReqSngIvtr) -> [CurrMeasGainReadReqSngIvtr]
  ES200B_CurrMeas/15(CurrMeasGainWrReqSngIvtr) -> [CurrMeasGainWrReqSngIvtr]
  ES200B_CurrMeas/16(CurrMeasOffsReadReqSngIvtr) -> [CurrMeasOffsReadReqSngIvtr]
  ES200B_CurrMeas/17(CurrMeasOffsWrReqSngIvtr) -> [CurrMeasOffsWrReqSngIvtr]
  [DiagcStsIvtr1Inactv] -> ES209B_CurrMeasCorrln/1(DiagcStsIvtr1Inactv)
  ES200B_CurrMeas/5(MotCtrlMotCurrCorrdA) -> ES209B_CurrMeasCorrln/2(MotCurrCorrdA), ES208A_CurrMeasArbn/3(MotCtrlMotCurrCorrdA)
  ES200B_CurrMeas/6(MotCtrlMotCurrCorrdB) -> ES209B_CurrMeasCorrln/3(MotCurrCorrdB), ES208A_CurrMeasArbn/4(MotCtrlMotCurrCorrdB)
  ES200B_CurrMeas/7(MotCtrlMotCurrCorrdC) -> ES209B_CurrMeasCorrln/4(MotCurrCorrdC), ES208A_CurrMeasArbn/5(MotCtrlMotCurrCorrdC)
  [MotCurrEolCalSt] -> ES209B_CurrMeasCorrln/5(MotCurrEolCalSt)
  [MotCurrQlfr1] -> ES209B_CurrMeasCorrln/6(MotCurrQlfr1)
  ES200B_CurrMeas/8(MotCtrlMotCurrRollgCntr1) -> ES209B_CurrMeasCorrln/7(MotCurrRollgCntr1), ES208A_CurrMeasArbn/11(MotCtrlMotCurrRollgCntr1)
  [SysSt] -> ES209B_CurrMeasCorrln/8(SysSt)
  [FltInj_u08] -> ES209B_CurrMeasCorrln/9(FltInj_u08)
  [GetNtcQlfrSts10] -> ES209B_CurrMeasCorrln/10(GetNtcQlfrSts)
  [SetNtcSts10] -> ES209B_CurrMeasCorrln/11(SetNtcSts)
  ES209B_CurrMeasCorrln/2(CurrMeasIdptSig) -> [CurrMeasIdptSig]
  ES209B_CurrMeasCorrln/3(CurrMotSumABC) -> [CurrMotSumABC]

== system Ford_T3T6_ArchCnctnDigrm/Monitor System/Measured Signals/ProcessHandwheelTorqueSignal ==
  note: ASIL D
  note: ASIL D
  note: ASIL D
  note: ASIL D
  note: ASIL D
  note: ASIL D
  CM660A_HwTq1Meas : Subsystem  Tag=1.10.0  Description=HandWheel Torque Sensor 1 Measurement
      settings: AttributesFormatString=Version: %<Tag>
  CM690D_HwTq8Meas : Subsystem  Tag=2.1.0  Description=Handwheel Torque 8 Measurement function using SENT protocol
      settings: AttributesFormatString=Version: %<Tag>
  ES224A_HwTq9Meas : Subsystem  Tag=1.7.0  Description=HwTq9Meas funtion shall compute handwheel torque by decoding the SENT protocol based on the timestamps provided by the GTM
      settings: AttributesFormatString=Version: %<Tag>
  ES225A_HwTq10Meas : Subsystem  Tag=1.8.0  Description=HwTq10Meas funtion shall compute handwheel torque by decoding the SENT protocol based on the timestamps provided by the GTM
      settings: AttributesFormatString=Version: %<Tag>
  ES228C_HwTqArbn : Subsystem  Tag=1.1.0  Description="Arbitration between multiple trq sensors and calculation of handwheel torque.  This version is unique in that is works with up to 4 unique HwTq signals.  There is no channel or pairs of torque signals concept."
      settings: AttributesFormatString=Version: %<Tag>
  ES229C_HwTqCorrln : Subsystem  Tag=1.0.0  Description="Function is responsible for immediate and long term correlation checks on the torque sensor signals.  This variant treats all of the input HwTq signals individually."
      settings: AttributesFormatString=Version: %<Tag>
  HwTq : Outport
  tag scope: HwTq10=global, HwTq10MeasHwTq10AutTrim=global, HwTq10MeasHwTq10ClrTrim=global, HwTq10MeasHwTq10ReadTrim=global, HwTq10MeasHwTq10TrimPrfmdSts=global, HwTq10MeasHwTq10WrTrim=global, HwTq10Qlfr=global, HwTq10RollgCntr=global, HwTq1=global, HwTq1MeasHwTq1AutTrim=global, HwTq1MeasHwTq1ClrTrim=global, HwTq1MeasHwTq1ReadTrim=global, HwTq1MeasHwTq1TrimPrfmdSts=global, HwTq1MeasHwTq1WrTrim=global, HwTq1MeasTrigStrt=global, HwTq1Qlfr=global, HwTq1RollgCntr=global, HwTq8=global, HwTq8AutTrim=global, HwTq8ClrTrim=global, HwTq8Qlfr=global, HwTq8ReadTrim=global, HwTq8RollgCntr=global, HwTq8TrigStrt=global, HwTq8TrimPrfmdSts=global, HwTq8WrTrim=global, HwTq9=global, HwTq9MeasHwTq9AutTrim=global, HwTq9MeasHwTq9ClrTrim=global, HwTq9MeasHwTq9ReadTrim=global, HwTq9MeasHwTq9TrimPrfmdSts=global, HwTq9MeasHwTq9WrTrim=global, HwTq9Qlfr=global, HwTq9RollgCntr=global, HwTqArbn=global, HwTqIdptSig=global, RackLimrCcwEotSig1=global, RackLimrCcwEotSig8=global, RackLimrCwEotSig1=global, RackLimrCwEotSig8=global, RackLimrEotSig1Avl=global, RackLimrEotSig8Avl=global
  wires:
  CM660A_HwTq1Meas/2(HwTq1Qlfr) -> ES229C_HwTqCorrln/5(HwTqBQlfr), [HwTq1Qlfr]
  CM660A_HwTq1Meas/3(HwTq1RollgCntr) -> ES229C_HwTqCorrln/6(HwTqBRollgCntr), [HwTq1RollgCntr]
  CM690D_HwTq8Meas/1(HwTq8) -> ES229C_HwTqCorrln/1(HwTqA), [HwTq8]
  CM690D_HwTq8Meas/2(HwTq8Qlfr) -> ES229C_HwTqCorrln/2(HwTqAQlfr), [HwTq8Qlfr]
  CM690D_HwTq8Meas/3(HwTq8RollgCntr) -> [HwTq8RollgCntr], ES229C_HwTqCorrln/3(HwTqARollgCntr)
  [HwTqBPolarity] -> CM660A_HwTq1Meas/1(HwTq1Polarity)
  [GetNtcQlfrSts10] -> CM660A_HwTq1Meas/2(GetNtcQlfrSts)
  [GetRefTmr1MicroSec32bit] -> CM660A_HwTq1Meas/3(GetRefTmr1MicroSec32bit)
  [GetTiSpan1MicroSec32bit] -> CM660A_HwTq1Meas/4(GetTiSpan1MicroSec32bit)
  [NvMProxy_SetRamBlockStatus] -> CM660A_HwTq1Meas/5(HwTq1Offs_SetRamBlockStatus)
  [IoHwAb_SetFctPrphlHwTq1] -> CM660A_HwTq1Meas/6(IoHwAb_SetFctPrphlHwTq1)
  [SetNtcSts10] -> CM660A_HwTq1Meas/7(SetNtcSts)
  CM660A_HwTq1Meas/4(RackLimrCcwEotSig1) -> [RackLimrCcwEotSig1]
  CM660A_HwTq1Meas/5(RackLimrCwEotSig1) -> [RackLimrCwEotSig1]
  CM660A_HwTq1Meas/6(RackLimrEotSig1Avl) -> [RackLimrEotSig1Avl]
  CM660A_HwTq1Meas/7(HwTq1MeasHwTq1AutTrim) -> [HwTq1MeasHwTq1AutTrim]
  CM660A_HwTq1Meas/8(HwTq1MeasHwTq1ClrTrim) -> [HwTq1MeasHwTq1ClrTrim]
  CM660A_HwTq1Meas/9(HwTq1MeasHwTq1ReadTrim) -> [HwTq1MeasHwTq1ReadTrim]
  CM660A_HwTq1Meas/10(HwTq1MeasHwTq1TrimPrfmdSts) -> [HwTq1MeasHwTq1TrimPrfmdSts]
  CM660A_HwTq1Meas/11(HwTq1MeasHwTq1WrTrim) -> [HwTq1MeasHwTq1WrTrim]
  CM660A_HwTq1Meas/12(HwTq1MeasTrigStrt) -> [HwTq1MeasTrigStrt]
  [HwTq8] -> ES228C_HwTqArbn/1(HwTqA)
  [HwTq8Qlfr] -> ES228C_HwTqArbn/2(HwTqAQlfr)
  [HwTq8RollgCntr] -> ES228C_HwTqArbn/3(HwTqARollgCntr)
  [HwTq1] -> ES228C_HwTqArbn/4(HwTqB)
  [HwTq1Qlfr] -> ES228C_HwTqArbn/5(HwTqBQlfr)
  [HwTq1RollgCntr] -> ES228C_HwTqArbn/6(HwTqBRollgCntr)
  [HwTq9] -> ES228C_HwTqArbn/7(HwTqC)
  [HwTq9Qlfr] -> ES228C_HwTqArbn/8(HwTqCQlfr)
  [HwTq9RollgCntr] -> ES228C_HwTqArbn/9(HwTqCRollgCntr)
  ES229C_HwTqCorrln/1(HwTqCorrlnSts) -> ES228C_HwTqArbn/10(HwTqCorrlnSts)
  [HwTq10] -> ES228C_HwTqArbn/11(HwTqD)
  [HwTq10Qlfr] -> ES228C_HwTqArbn/12(HwTqDQlfr)
  [HwTq10RollgCntr] -> ES228C_HwTqArbn/13(HwTqDRollgCntr)
  [FltInj_f32] -> ES228C_HwTqArbn/14(FltInj_f32)
  CM660A_HwTq1Meas/1(HwTq1) -> ES229C_HwTqCorrln/4(HwTqB), [HwTq1]
  [FltInj_u08] -> ES229C_HwTqCorrln/13(FltInj_u08)
  [GetNtcQlfrSts10] -> ES229C_HwTqCorrln/14(GetNtcQlfrSts)
  [SetNtcSts10] -> ES229C_HwTqCorrln/15(SetNtcSts)
  ES229C_HwTqCorrln/2(HwTqIdptSig) -> [HwTqIdptSig]
  [HwTqCPolarity] -> ES224A_HwTq9Meas/1(HwTq9Polarity)
  [GetNtcQlfrSts] -> ES224A_HwTq9Meas/2(GetNtcQlfrSts)
  [GtmGetSent0Data] -> ES224A_HwTq9Meas/3(GtmGetSent0Data)
  [NvMProxy_GetErrorStatus] -> ES224A_HwTq9Meas/4(HwTq9Offs_GetErrorStatus)
  [NvMProxy_SetRamBlockStatus] -> ES224A_HwTq9Meas/5(HwTq9Offs_SetRamBlockStatus)
  [SetNtcSts10] -> ES224A_HwTq9Meas/6(SetNtcSts)
  [SetNtcStsAndSnpshtData10] -> ES224A_HwTq9Meas/7(SetNtcStsAndSnpshtData)
  ES224A_HwTq9Meas/1(HwTq9) -> [HwTq9], ES229C_HwTqCorrln/7(HwTqC)
  ES224A_HwTq9Meas/2(HwTq9Qlfr) -> [HwTq9Qlfr], ES229C_HwTqCorrln/8(HwTqCQlfr)
  ES224A_HwTq9Meas/3(HwTq9RollgCntr) -> [HwTq9RollgCntr], ES229C_HwTqCorrln/9(HwTqCRollgCntr)
  ES224A_HwTq9Meas/4(HwTq9MeasHwTq9AutTrim) -> [HwTq9MeasHwTq9AutTrim]
  ES224A_HwTq9Meas/5(HwTq9MeasHwTq9ClrTrim) -> [HwTq9MeasHwTq9ClrTrim]
  ES224A_HwTq9Meas/6(HwTq9MeasHwTq9ReadTrim) -> [HwTq9MeasHwTq9ReadTrim]
  ES224A_HwTq9Meas/7(HwTq9MeasHwTq9TrimPrfmdSts) -> [HwTq9MeasHwTq9TrimPrfmdSts]
  ES224A_HwTq9Meas/8(HwTq9MeasHwTq9WrTrim) -> [HwTq9MeasHwTq9WrTrim]
  [HwTqDPolarity] -> ES225A_HwTq10Meas/1(HwTq10Polarity)
  [GetNtcQlfrSts10] -> ES225A_HwTq10Meas/2(GetNtcQlfrSts)
  [GtmGetSent1Data] -> ES225A_HwTq10Meas/3(GtmGetSent1Data)
  [NvMProxy_GetErrorStatus] -> ES225A_HwTq10Meas/4(HwTq10Offs_GetErrorStatus)
  [NvMProxy_SetRamBlockStatus] -> ES225A_HwTq10Meas/5(HwTq10Offs_SetRamBlockStatus)
  [SetNtcSts10] -> ES225A_HwTq10Meas/6(SetNtcSts)
  [SetNtcStsAndSnpshtData10] -> ES225A_HwTq10Meas/7(SetNtcStsAndSnpshtData)
  ES225A_HwTq10Meas/2(HwTq10Qlfr) -> [HwTq10Qlfr], ES229C_HwTqCorrln/11(HwTqDQlfr)
  ES225A_HwTq10Meas/3(HwTq10RollgCntr) -> [HwTq10RollgCntr], ES229C_HwTqCorrln/12(HwTqDRollgCntr)
  ES225A_HwTq10Meas/4(HwTq10MeasHwTq10AutTrim) -> [HwTq10MeasHwTq10AutTrim]
  ES225A_HwTq10Meas/5(HwTq10MeasHwTq10ClrTrim) -> [HwTq10MeasHwTq10ClrTrim]
  ES225A_HwTq10Meas/6(HwTq10MeasHwTq10ReadTrim) -> [HwTq10MeasHwTq10ReadTrim]
  ES225A_HwTq10Meas/7(HwTq10MeasHwTq10TrimPrfmdSts) -> [HwTq10MeasHwTq10TrimPrfmdSts]
  ES225A_HwTq10Meas/8(HwTq10MeasHwTq10WrTrim) -> [HwTq10MeasHwTq10WrTrim]
  ES225A_HwTq10Meas/1(HwTq10) -> [HwTq10], ES229C_HwTqCorrln/10(HwTqD)
  ES228C_HwTqArbn/1(HwTq) -> HwTq/1, [HwTqArbn]
  [HwTqAPolarity] -> CM690D_HwTq8Meas/1(HwTq8Polarity)
  [CnvSnpshtData_u08] -> CM690D_HwTq8Meas/2(CnvSnpshtData_u08)
  [FltInj_f32] -> CM690D_HwTq8Meas/3(FltInj_f32)
  [FltInj_u08] -> CM690D_HwTq8Meas/4(FltInj_u08)
  [GetNtcQlfrSts10] -> CM690D_HwTq8Meas/5(GetNtcQlfrSts)
  [GetRefTmr1MicroSec32bit] -> CM690D_HwTq8Meas/6(GetRefTmr1MicroSec32bit)
  [GetTiSpan1MicroSec32bit] -> CM690D_HwTq8Meas/7(GetTiSpan1MicroSec32bit)
  [NvMProxy_SetRamBlockStatus] -> CM690D_HwTq8Meas/8(HwTq8Offs_SetRamBlockStatus)
  [IoHwAb_SetFctPrphlHwTq2] -> CM690D_HwTq8Meas/9(IoHwAb_SetFctPrphlHwTq8)
  [SetNtcStsAndSnpshtData10] -> CM690D_HwTq8Meas/10(SetNtcStsAndSnpshtData)
  CM690D_HwTq8Meas/4(RackLimrCcwEotSig8) -> [RackLimrCcwEotSig8]
  CM690D_HwTq8Meas/5(RackLimrCwEotSig8) -> [RackLimrCwEotSig8]
  CM690D_HwTq8Meas/6(RackLimrEotSig8Avl) -> [RackLimrEotSig8Avl]
  CM690D_HwTq8Meas/7(HwTq8AutTrim) -> [HwTq8AutTrim]
  CM690D_HwTq8Meas/8(HwTq8ClrTrim) -> [HwTq8ClrTrim]
  CM690D_HwTq8Meas/9(HwTq8ReadTrim) -> [HwTq8ReadTrim]
  CM690D_HwTq8Meas/10(HwTq8TrigStrt) -> [HwTq8TrigStrt]
  CM690D_HwTq8Meas/11(HwTq8TrimPrfmdSts) -> [HwTq8TrimPrfmdSts]
  CM690D_HwTq8Meas/12(HwTq8WrTrim) -> [HwTq8WrTrim]

== system Ford_T3T6_ArchCnctnDigrm/States and Modes/SystemStartUpState/ES003C_PwrDiscnct ==
  BattVltg : Inport
  BattVltgAdcFaild : Inport  Port=2
  BattVltgSwd1 : Inport  Port=3
  ChrgPmpDiag : Inport  Port=4
  ChrgPmpDiagAdcFaild : Inport  Port=5
  MotVelMrf : Inport  Port=6
  PwrDiscnctSwtDiag : Inport  Port=7
  StrtUpSt : Inport  Port=8
  SysSt : Inport  Port=9
  CnvSnpshtData_f32 : Inport  Port=10
  GetNtcQlfrSts : Inport  Port=11
  SetNtcStsAndSnpshtData : Inport  Port=12
  Ivtr1PwrDiscnctFltSts : Outport
  PwrDiscnctATestCmpl : Outport  Port=2
  PwrDiscnctBTestCmpl : Outport  Port=3

== system Ford_T3T6_ArchCnctnDigrm/States and Modes/SystemStartUpState/ES004A_PwrUpSeq ==
  CodFlsCrcChkCmpl : Inport
  CurrMeasWrmIninTestCmpl : Inport  Port=2
  MotDrvr0IninTestCmpl : Inport  Port=3
  MotDrvr1IninTestCmpl : Inport  Port=4
  PhaDiscnctWrmIninTestCmpl : Inport  Port=5
  PwrDiscnctATestCmpl : Inport  Port=6
  PwrDiscnctBTestCmpl : Inport  Port=7
  SysSt : Inport  Port=8
  TmplMonIninTestCmpl : Inport  Port=9
  IoHwAb_SetGpioPwrTurnOffCtrl : Inport  Port=10
  StrtUpSt : Outport
  SysStWrmIninCmpl : Outport  Port=2
  PwrTurnOffCtrl : Outport  Port=3

== system Ford_T3T6_ArchCnctnDigrm/States and Modes/SystemStartUpState/ES005C_TmplMonr ==
  StrtUpSt : Inport
  SysSt : Inport  Port=2
  Spi_GetSequenceResult : Inport  Port=3
  Call_Spi_AsyncTransmit : Inport  Port=4
  CtrlErrOut : Inport  Port=5
  GetRefTmr1MicroSec32bit : Inport  Port=6
  GetTiSpan1MicroSec32bit : Inport  Port=7
  IoHwAb_GetGpioPwrOutpEnaFb : Inport  Port=8
  IoHwAb_SetGpioTmplMonrWdg : Inport  Port=9
  SetNtcSts : Inport  Port=10
  Spi_ReadIB : Inport  Port=11
  Spi_WriteIB : Inport  Port=12
  TmplMonrIninTestCmpl : Outport

== system Ford_T3T6_ArchCnctnDigrm/States and Modes/SystemStartUpState/ES008A_PwrSply ==
  SysSt : Inport
  Spi_GetSequenceResult : Inport  Port=2
  Call_Spi_AsyncTransmit : Inport  Port=3
  SetNtcSts : Inport  Port=4
  Spi_ReadIB : Inport  Port=5
  Spi_WriteIB : Inport  Port=6

== system Ford_T3T6_ArchCnctnDigrm/States and Modes/SystemStartUpState/ES108A_ShtdwnMech ==
  DiagcStsIvtr1Inactv : Inport
  StrtUpSt : Inport  Port=2
  IoHwAb_SetGpioSysFlt2A : Inport  Port=3

== system Ford_T3T6_ArchCnctnDigrm/States and Modes/SystemStartUpState/ES311A_GateDrv0Ctrl ==
  Ivtr1PwrDiscnctFltSts : Inport
  PhaOnTiMeasdA : Inport  Port=2
  PhaOnTiMeasdB : Inport  Port=3
  PhaOnTiMeasdC : Inport  Port=4
  PhaOnTiSumA : Inport  Port=5
  PhaOnTiSumB : Inport  Port=6
  PhaOnTiSumC : Inport  Port=7
  StrtUpSt : Inport  Port=8
  SysSt : Inport  Port=9
  Call_Spi_AsyncTransmit : Inport  Port=10
  GetNtcQlfrSts : Inport  Port=11
  IoHwAb_GetGpioMotDrvr0Diag : Inport  Port=12
  IoHwAb_SetGpioGateDrv0Rst : Inport  Port=13
  IoHwAb_SetGpioSysFlt2A : Inport  Port=14
  SetNtcSts : Inport  Port=15
  SetNtcStsAndSnpshtData : Inport  Port=16
  Spi_GetSequenceResult : Inport  Port=17
  Spi_ReadIB : Inport  Port=18
  Spi_WriteIB : Inport  Port=19
  DiagcStsIvtr1Inactv : Outport
  IvtrFetFltPha : Outport  Port=2
  IvtrFetFltTyp : Outport  Port=3
  MotDrvErrA : Outport  Port=4
  MotDrvErrB : Outport  Port=5
  MotDrvErrC : Outport  Port=6
  MotDrvr0IninTestCmpl : Outport  Port=7

== system Ford_T3T6_ArchCnctnDigrm/Vector Components Base Software/COM/AR001ACom_Com ==

== system Ford_T3T6_ArchCnctnDigrm/Vector Components Base Software/COM/AR001AIPduM_IPduM ==

== system Ford_T3T6_ArchCnctnDigrm/Vector Components Base Software/COM/AR001APduR_PduR ==

== system Ford_T3T6_ArchCnctnDigrm/Vector Components Base Software/DIAG/AR001ADcm_Dcm ==

== system Ford_T3T6_ArchCnctnDigrm/Vector Components Base Software/DIAG/AR001ADem_Dem ==
  Dem_ClearDTC : Outport
  Dem_GetDTCOfEvent : Outport  Port=2
  Dem_GetEventStatus : Outport  Port=3
  Dem_GetIndicatorStatus : Outport  Port=4
  Dem_ReportErrorStatus : Outport  Port=5
  Dem_SetEventStatus : Outport  Port=6

== system Ford_T3T6_ArchCnctnDigrm/Vector Components Base Software/IO/AR001A_IoHwAb ==
  IoHwAb_GetGpioEcuIdnPin1 : Outport
  IoHwAb_GetGpioEcuIdnPin2 : Outport  Port=2
  IoHwAb_GetGpioMcuEna : Outport  Port=3
  IoHwAb_GetGpioMotDrvr0Diag : Outport  Port=4
  IoHwAb_GetGpioPwrOutpEnaFb : Outport  Port=5
  IoHwAb_SetFctGpioPhaALowrCmd : Outport  Port=6
  IoHwAb_SetFctGpioPhaAUpprCmd : Outport  Port=7
  IoHwAb_SetFctGpioPhaBLowrCmd : Outport  Port=8
  IoHwAb_SetFctGpioPhaBUpprCmd : Outport  Port=9
  IoHwAb_SetFctGpioPhaCLowrCmd : Outport  Port=10
  IoHwAb_SetFctGpioPhaCUpprCmd : Outport  Port=11
  IoHwAb_SetFctPrphlHwAg1 : Outport  Port=12
  IoHwAb_SetFctPrphlHwTq1 : Outport  Port=13
  IoHwAb_SetFctPrphlHwTq2 : Outport  Port=14
  IoHwAb_SetFctPrphlPhaALowrCmd : Outport  Port=15
  IoHwAb_SetFctPrphlPhaAUpprCmd : Outport  Port=16
  IoHwAb_SetFctPrphlPhaBLowrCmd : Outport  Port=17
  IoHwAb_SetFctPrphlPhaBUpprCmd : Outport  Port=18
  IoHwAb_SetFctPrphlPhaCLowrCmd : Outport  Port=19
  IoHwAb_SetFctPrphlPhaCUpprCmd : Outport  Port=20
  IoHwAb_SetGpioGateDrv0Rst : Outport  Port=21
  IoHwAb_SetGpioPhaALowrCmd : Outport  Port=22
  IoHwAb_SetGpioPhaAUpprCmd : Outport  Port=23
  IoHwAb_SetGpioPhaBLowrCmd : Outport  Port=24
  IoHwAb_SetGpioPhaBUpprCmd : Outport  Port=25
  IoHwAb_SetGpioPhaCLowrCmd : Outport  Port=26
  IoHwAb_SetGpioPhaCUpprCmd : Outport  Port=27
  IoHwAb_SetGpioPwrTurnOffCtrl : Outport  Port=28
  IoHwAb_SetGpioSysFlt2A : Outport  Port=29
  IoHwAb_SetGpioTmplMonrWdg : Outport  Port=30

== system Ford_T3T6_ArchCnctnDigrm/Vector Components Base Software/MCAL/AR001AMcu_Mcu ==
  Mcu_PerformReset : Outport

== system Ford_T3T6_ArchCnctnDigrm/Vector Components Base Software/MCAL/AR001AWdg_Wdg ==

== system Ford_T3T6_ArchCnctnDigrm/Vector Components Base Software/MEM/AR001AFee_Fee ==

== system Ford_T3T6_ArchCnctnDigrm/Vector Components Base Software/MEM/AR001AMemIf_MemIf ==

== system Ford_T3T6_ArchCnctnDigrm/Vector Components Base Software/MEM/AR001ANvM_NvM ==
  NvM_CancelWriteAll : Outport
  NvM_GetErrorStatus : Outport  Port=2
  NvM_ReadAll : Outport  Port=3
  NvM_ReadBlock : Outport  Port=4
  NvM_SetRamBlockStatus : Outport  Port=5
  NvM_WriteAll : Outport  Port=6
  NvM_WriteBlock : Outport  Port=7

== system Ford_T3T6_ArchCnctnDigrm/Vector Components Base Software/SYS/AR001ABswM_BswM ==
  BswM_RequestMode : Outport

== system Ford_T3T6_ArchCnctnDigrm/Vector Components Base Software/SYS/AR001AComM_ComM ==
  ComM_RequestComMode : Outport

== system Ford_T3T6_ArchCnctnDigrm/Vector Components Base Software/SYS/AR001ADet_Det ==

== system Ford_T3T6_ArchCnctnDigrm/Vector Components Base Software/SYS/AR001AWdgIf_WdgIf ==

== system Ford_T3T6_ArchCnctnDigrm/Vector Components Base Software/SYS/AR001AWdgM_WdgM ==
  PortDefinedArgument_CheckpointReached : Outport
  WdgM_ActivateSupervisionEntity : Outport  Port=2
  WdgM_CheckpointReached : Outport  Port=3
  WdgM_DeactivateSupervisionEntity : Outport  Port=4

== system Ford_T3T6_ArchCnctnDigrm/Vehicle Com/Rx Messages/Acc Pedal Posn ==
  note: From COM
  note: From COM
  ApedPosPcActl_D_Qf : Ground
  ApedPos_Pc_ActlArb : Ground
  EngAout_N_Actl : Ground
  MM062A_FordMsg204BusHiSpd : Subsystem  Tag=1.0.0  Description=The purpose of the Ford Message 204 Bus High Speed function is toprovide the Electric Power Steering system with signal values forthe Trailer Back Up Assist function from CAN. The Ford Message 204function will perform the missing message and signal invalid diagnostics and provide validity signals for the received message and signal values.
      settings: AttributesFormatString=Version: %<Tag>
  tag scope: FordMsg204HiSpdBusClrDiagcSrv=global, FordMsg204HiSpdBusSerlComInpDi=global, FordVehAccrPedlPosnStsQlyFac=global, FordVehAccrPedlPosnStsQlyFacRaw=global, FordVehAccrPedlPosnStsRaw=global, FordVehAccrPedlPosnStsVld=global, FordVehEngSpdRaw=global, FordVehEngSpdVld=global
  wires:
  ApedPos_Pc_ActlArb/1 -> MM062A_FordMsg204BusHiSpd/1(AccrPedlPosnSts)
  ApedPosPcActl_D_Qf/1 -> MM062A_FordMsg204BusHiSpd/2(AccrPedlPosnStsQlyFac)
  [FordCanDtcInhb] -> MM062A_FordMsg204BusHiSpd/3(CanDtcInhb)
  EngAout_N_Actl/1 -> MM062A_FordMsg204BusHiSpd/4(EngSpd)
  [FordEpsLifeCycMod] -> MM062A_FordMsg204BusHiSpd/5(EpsLifeCycMod)
  [FordTrlrBackupAssiEnad] -> MM062A_FordMsg204BusHiSpd/6(TrlrBackUpAssiEnad)
  [GetRefTmr100MicroSec32bit] -> MM062A_FordMsg204BusHiSpd/7(GetRefTmr100MicroSec32bit)
  [GetTiSpan100MicroSec32bit] -> MM062A_FordMsg204BusHiSpd/8(GetTiSpan100MicroSec32bit)
  [SetNtcSts] -> MM062A_FordMsg204BusHiSpd/9(SetNtcSts)
  MM062A_FordMsg204BusHiSpd/1(FordVehAccrPedlPosnStsQlyFac) -> [FordVehAccrPedlPosnStsQlyFac]
  MM062A_FordMsg204BusHiSpd/2(FordVehAccrPedlPosnStsQlyFacRaw) -> [FordVehAccrPedlPosnStsQlyFacRaw]
  MM062A_FordMsg204BusHiSpd/3(FordVehAccrPedlPosnStsRaw) -> [FordVehAccrPedlPosnStsRaw]
  MM062A_FordMsg204BusHiSpd/4(FordVehAccrPedlPosnStsVld) -> [FordVehAccrPedlPosnStsVld]
  MM062A_FordMsg204BusHiSpd/5(FordVehEngSpdRaw) -> [FordVehEngSpdRaw]
  MM062A_FordMsg204BusHiSpd/6(FordVehEngSpdVld) -> [FordVehEngSpdVld]
  MM062A_FordMsg204BusHiSpd/7(FordMsg204HiSpdBusClrDiagcSrv) -> [FordMsg204HiSpdBusClrDiagcSrv]
  MM062A_FordMsg204BusHiSpd/8(FordMsg204HiSpdBusSerlComInpDi) -> [FordMsg204HiSpdBusSerlComInpDi]
